simulink model "Software_Pacing"  (R2020a)
settings: Solver=FixedStepAuto  StartTime=0.0  StopTime=15.0  FixedStep=1e-3  RelTol=1e-3  EnableMultiTasking=on
undefined symbols (not defined in the file): D10, D11, D12, D2, D4, D5, D7, D8, D9, PTA0, PTA2, PTB23, PTB9, PTC3, PTC4, PTD0, PTD2, PTD3
libraries: frdmk64flib x9
settings Model: ExtModeTrigDuration=5  Creator=Costco Member  LastModifiedBy=Costco Member
settings OptimizationCC: EnhancedBackFolding=on  PassReuseOutputArgsAs=Individual arguments  ZeroExternalMemoryAtStartup=off  ZeroInternalMemoryAtStartup=off  MaxStackSize=64  OptimizeBlockOrder=speed  DifferentSizesBufferReuse=on  OptimizationCustomize=off  EfficientTunableParamExpr=on
settings DebuggingCC: ParameterTunabilityLossMsg=error
settings HardwareCC: ProdBitPerPointer=32  ProdBitPerSizeT=32  ProdBitPerPtrDiffT=32  ProdLargestAtomicInteger=Long  ProdLargestAtomicFloat=Double  ProdWordSize=32  ProdHWDeviceType=ARM Compatible->ARM Cortex
settings SFSimCC: MATLABDynamicMemAlloc=off
settings RTWCC: SystemTargetFile=ert.tlc  HardwareBoard=NXP FRDM-K64F  TemplateMakefile=ert_default_tmf  Toolchain=GNU Tools for ARM Embedded Processors
settings CodeAppCC: ForceParamTrailComments=on  IgnoreCustomStorageClasses=off  OperatorAnnotations=on  SimulinkDataObjDesc=on  SFDataObjDesc=on  InsertBlockDesc=on

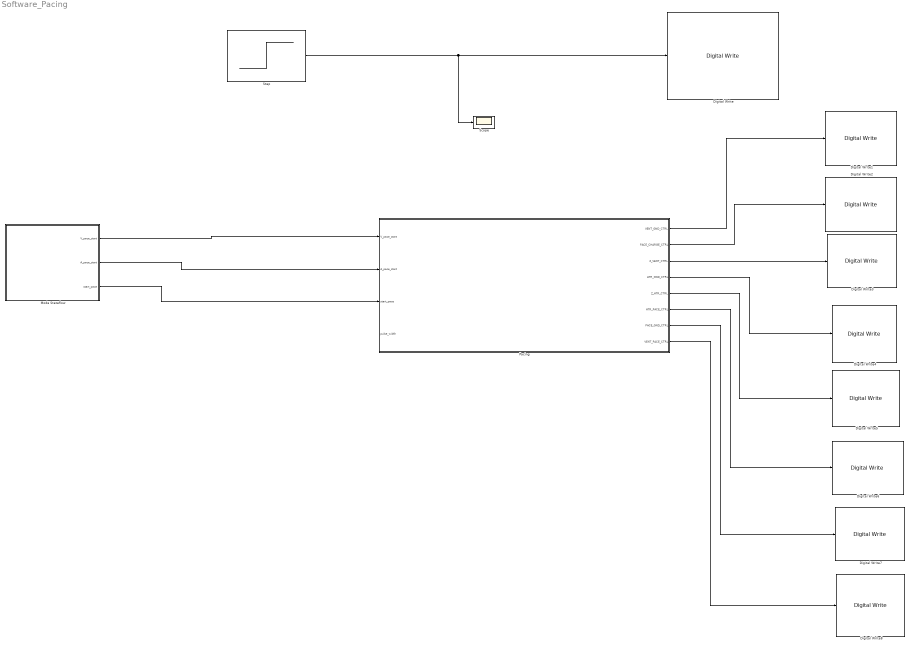
== system Software_Pacing ==
  Digital Write : frdmk64flib/Digital Write  Whichpin=PTA2 (D5)
  Digital Write1 : frdmk64flib/Digital Write  Whichpin=PTD3 (D12)
  Digital Write2 : frdmk64flib/Digital Write  Whichpin=PTB9 (D2)
  Digital Write3 : frdmk64flib/Digital Write  Whichpin=PTC3 (D7)
  Digital Write4 : frdmk64flib/Digital Write  Whichpin=PTD2 (D11)
  Digital Write5 : frdmk64flib/Digital Write  Whichpin=PTB23 (D4)
  Digital Write6 : frdmk64flib/Digital Write  Whichpin=PTA0 (D8)
  Digital Write7 : frdmk64flib/Digital Write  Whichpin=PTD0 (D10)
  Digital Write8 : frdmk64flib/Digital Write  Whichpin=PTC4 (D9)
  Mode Stateflow : Stateflow chart  TreatAsAtomicUnit=on
  Pacing : Stateflow chart  TreatAsAtomicUnit=on
  Scope : Scope
  Step : Step  Time=5  SampleTime=5
  wires:
  Step/1 -> Scope/1, Digital Write/1
  Mode Stateflow/1(V_pace_start) -> Pacing/1(V_pace_start)
  Mode Stateflow/2(A_pace_start) -> Pacing/2(A_pace_start)
  Pacing/1(VENT_GND_CTRL) -> Digital Write1/1
  Pacing/2(PACE_CHARGE_CTRL) -> Digital Write2/1
  Pacing/3(Z_VENT_CTRL) -> Digital Write3/1
  Pacing/4(ATR_GND_CTRL) -> Digital Write4/1
  Pacing/5(Z_ATR_CTRL) -> Digital Write5/1
  Pacing/6(ATR_PACE_CTRL) -> Digital Write6/1
  Pacing/7(PACE_GND_CTRL) -> Digital Write7/1
  Pacing/8(VENT_PACE_CTRL) -> Digital Write8/1
  Mode Stateflow/3(start_pace) -> Pacing/3(start_pace)

== stateflow chart Software_Pacing/Mode Stateflow ==
  state AOO
    entry:
    A_pace_start=true;
    V_pace_start=false;
    start_pace=true;
  state VOO
    entry:
    A_pace_start=false;
    V_pace_start=true;
    start_pace=true;
  (default) -> AOO
  AOO -> VOO
  VOO -> AOO
  data: V_pace_start output boolean; A_pace_start output boolean; start_pace output boolean

== stateflow chart Software_Pacing/Pacing ==
  state A_Pacing
    entry:
    PACE_CHARGE_CTRL=false;
    PACE_GND_CTRL=true;
    ATR_PACE_CTRL=true;
    ATR_GND_CTRL=false;
    Z_ATR_CTRL=false;
    Z_VENT_CTRL=false;
    VENT_GND_CTRL=false;
    VENT_PACE_CTRL=false;
  state V_Pacing
    entry:
    PACE_CHARGE_CTRL=false;
    PACE_GND_CTRL=true;
    ATR_PACE_CTRL=false;
    ATR_GND_CTRL=false;
    Z_ATR_CTRL=false;
    Z_VENT_CTRL=false;
    VENT_GND_CTRL=false;
    VENT_PACE_CTRL=true;
  state C22_Charge
    entry:
    PACE_GND_CTRL=false;
    VENT_PACE_CTRL=false;
    PACE_CHARGE_CTRL=true;
  state C21_Discharge_V
    entry:
    PACE_GND_CTRL=true;
    VENT_PACE_CTRL=false;
    Z_ATR_CTRL=false;
    Z_VENT_CTRL=false;
    ATR_PACE_CTRL=false;
    ATR_GND_CTRL=false;
    VENT_GND_CTRL=true;
  state C21_Discharge_A
    entry:
    PACE_GND_CTRL=true;
    VENT_PACE_CTRL=false;
    Z_ATR_CTRL=false;
    Z_VENT_CTRL=false;
    ATR_PACE_CTRL=false;
    ATR_GND_CTRL=true;
    VENT_GND_CTRL=false;
  (default) -> C22_Charge
  C22_Charge -> V_Pacing [order 1] : [V_pace_start==true && start_pace==true]
  C22_Charge -> A_Pacing [order 2] : [A_pace_start==true && start_pace==true]
  C21_Discharge_A -> C22_Charge
  C21_Discharge_V -> C22_Charge
  A_Pacing -> C21_Discharge_A : after(pulse_width,msec)
  V_Pacing -> C21_Discharge_V : after(pulse_width,msec)
  data: VENT_GND_CTRL output boolean; PACE_CHARGE_CTRL output boolean; Z_VENT_CTRL output boolean; ATR_GND_CTRL output boolean; Z_ATR_CTRL output boolean; ATR_PACE_CTRL output boolean; PACE_GND_CTRL output boolean; VENT_PACE_CTRL output boolean; V_pace_start input boolean; A_pace_start input boolean; start_pace input boolean; pulse_width input double
